simulink model "untitled"  (R2017a)
settings: Solver=VariableStepAuto  StartTime=0.0  StopTime=10.0  RelTol=1e-3
values from neighbouring files (symbols this model uses):
  tdot_2 = u(2)    [link_solver.m]
undefined symbols (not defined in the file or in its folder): theta2_stop, v_0, x_0
libraries: simulink x1
settings Model: Creator=rahul  LastModifiedBy=rahul

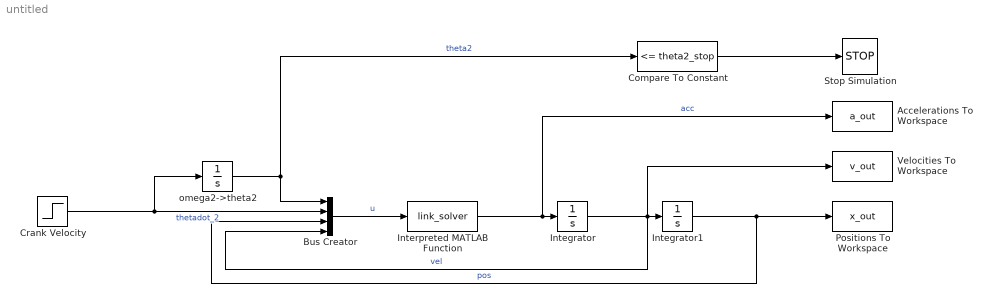
== system untitled ==
  Accelerations To Workspace : ToWorkspace  VariableName=a_out  SampleTime=-1
  Bus Creator : BusCreator  Inputs=4
  Compare To Constant : simulink/Logic and Bit Operations/Compare To Constant  relop=<=  const=theta2_stop  OutDataTypeStr=boolean
  Crank Velocity : Step  Time=0  After=tdot_2  SampleTime=0
  Integrator : Integrator  InitialCondition=v_0
  Integrator1 : Integrator  InitialCondition=x_0
  Interpreted MATLAB Function : MATLABFcn  MATLABFcn=link_solver
  Positions To Workspace : ToWorkspace  VariableName=x_out  SampleTime=-1
  Stop Simulation : Stop
  Velocities To Workspace : ToWorkspace  VariableName=v_out  SampleTime=-1
  omega2->theta2 : Integrator
  wires:
  Interpreted MATLAB Function/1 -> Accelerations To Workspace/1, Integrator/1  "acc"
  Integrator/1 -> Velocities To Workspace/1, Bus Creator/4, Integrator1/1  "vel"
  Bus Creator/1 -> Interpreted MATLAB Function/1  "u"
  Crank Velocity/1 -> omega2->theta2/1, Bus Creator/2  "thetadot_2"
  omega2->theta2/1 -> Compare To Constant/1, Bus Creator/1  "theta2"
  Integrator1/1 -> Positions To Workspace/1, Bus Creator/3  "pos"
  Compare To Constant/1 -> Stop Simulation/1
